simulink model "SMD_System"  (R2025b)
settings: Solver=VariableStepAuto  StartTime=0.0  StopTime=inf  MaxStep=0.01  RelTol=1e-3
undefined symbols (not defined in the file or in its folder): b
libraries: fl_lib x7, nesl_utility x3, fuzblock x1
settings Model: Creator=muham  LastModifiedBy=leffe
settings SolverCC: AlgebraicLoopSolver=TrustRegion
settings OptimizationCC: BlockReduction=off
settings DebuggingCC: UnconnectedInputMsg=warning  UnconnectedOutputMsg=warning  UnconnectedLineMsg=warning
settings ModelReferenceCC: EnableRefExpFcnMdlSchedulingChecks=on
settings SFSimCC: CustomCodeUndefinedFunction=UseInterfaceOnly
settings RTWCC: GPUComputeCapability=3.5
settings ExplorerConfigSet: SimMechanicsOpenEditorOnUpdate=off

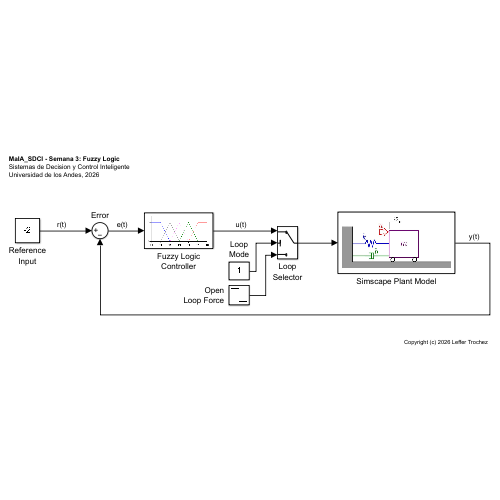
[thumbnail: Simulink's stored preview of the top-level diagram]
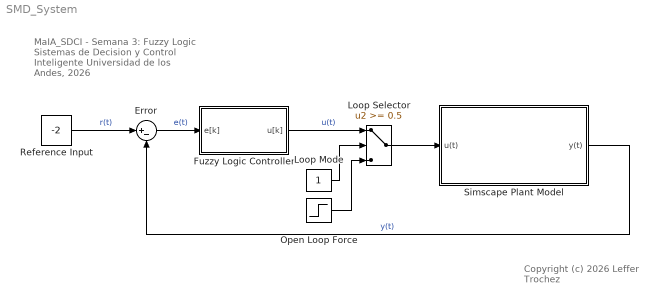
== system SMD_System ==
  note: Copyright (c) 2026 Leffer Trochez
  note: MaIA_SDCI - Semana 3: Fuzzy Logic
      | Sistemas de Decision y Control Inteligente
      | Universidad de los Andes, 2026
  Error : Sum  Inputs=|+-
  Fuzzy Logic Controller : Subsystem
      mask Display: image('fuzzy.png', [0,0,0,0,90,90]);
  Loop Mode : Constant
  Loop Selector : Switch  Threshold=0.5  SaturateOnIntegerOverflow=off  InputSameDT=off
  Open Loop Force : Step  Time=0.03  Before=500  After=0  SampleTime=0
  Reference Input : Constant  Value=-2  SampleTime=0
  Simscape Plant Model : Subsystem
      mask Display: image('Fig.png');
  wires:
  Error/1 -> Fuzzy Logic Controller/1(e[k])  "e(t)"
  Reference Input/1 -> Error/1  "r(t)"
  Simscape Plant Model/1(y(t)) -> Error/2  "y(t)"
  Fuzzy Logic Controller/1(u[k]) -> Loop Selector/1  "u(t)"
  Loop Mode/1 -> Loop Selector/2
  Open Loop Force/1 -> Loop Selector/3
  Loop Selector/1 -> Simscape Plant Model/1(u(t))

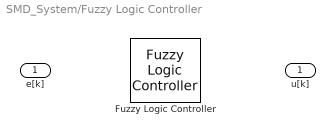
== system SMD_System/Fuzzy Logic Controller ==
  e[k] : Inport
  "Fuzzy Logic Controller " : fuzblock/Fuzzy Logic  Controller  FIS='tipper.fis'  OutputSampleNumber=101  DataType=double  UseLookupTable=off  NumBreakpoints=10  FuzzifiedInputs=off  RuleFiringStrengths=off  RuleOutputs=off  AggregatedOutputs=off  SimulateUsing=Interpreted execution  OutOfRangeInputValueMessage=warning  NoRuleFiredMessage=warning  EmptyOutputFuzzySetMessage=warning
  u[k] : Outport

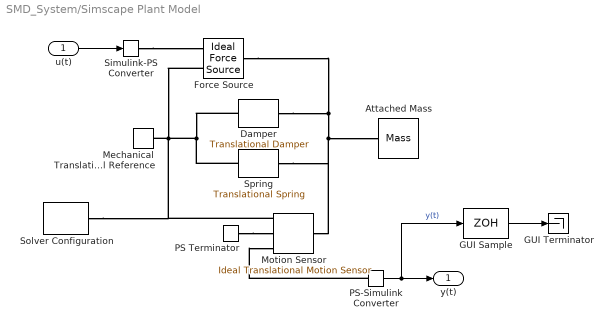
== system SMD_System/Simscape Plant Model ==
  u(t) : Inport
  Attached Mass : fl_lib/Mechanical/Translational Elements/Mass  mass=m kg  num_ports=foundation.enum.numPorts2.one  v_specify=off  v_priority=High  v=0 m/s  v_nominal_specify=off  v_nominal_value=1  v_nominal_unit=m/s  f_specify=off  f_priority=None  f=0 N  f_nominal_specify=off  f_nominal_value=1  f_nominal_unit=N
  Damper : fl_lib/Mechanical/Translational Elements/Translational Damper  D=b N/(m/s)  v_specify=off  v_priority=None  v=0 m/s  v_nominal_specify=off  v_nominal_value=1  v_nominal_unit=m/s  f_specify=off  f_priority=None  f=0 N  f_nominal_specify=off  f_nominal_value=1  f_nominal_unit=N
  Force Source : fl_lib/Mechanical/Mechanical Sources/Ideal Force Source
  GUI Terminator : Terminator
  GUI Sample : ZeroOrderHold  SampleTime=0.02
  Mechanical Translational Reference : fl_lib/Mechanical/Translational Elements/Mechanical Translational Reference
  Motion Sensor : fl_lib/Mechanical/Mechanical Sensors/Ideal Translational Motion Sensor  reference=foundation.enum.MeasurementReference.difference  acceleration_port=false  velocity_port=true  position_port=true  offset=0 m
  PS Terminator : fl_lib/Physical Signals/Sinks/PS Terminator
  PS-Simulink Converter : nesl_utility/PS-Simulink Converter  PhysicalDomain=network_engine_domain  SubClassName=ps_output  LeftPortType=input  RightPortType=output  PseudoPeriodic=off  Frequencies=[]  VectorFormat=1-D array  Unit=m  AffineConversion=off
  Simulink-PS Converter : nesl_utility/Simulink-PS Converter  PhysicalDomain=network_engine_domain  SubClassName=ps_input  LeftPortType=input  RightPortType=output  PseudoPeriodic=off  Frequencies=[]  NoiseDistribution=none  NoiseParameters=[]  Unit=N  AffineConversion=off  FilteringAndDerivatives=provide  SimscapeFilterOrder=1  InputFilterTimeConstant=0.001  UdotUserProvided=0
  Solver Configuration : nesl_utility/Solver Configuration  PhysicalDomain=network_engine_domain  SubClassName=solver  LeftPortType=input  RightPortType=generic  Tones=[]  Harmonics=[]  SimulateNoise=off  Profile=off  UseLocalSampling=off  EnableSwitchedLinearOptims=on  FrequencyDomain=off  UseCCode=off  RelTol=0.001  AbsTol=1e-06  MinStep=1e-09  ToWorkspace=off  RevertToSquareIcSolve=off  NumHomotopyIterations=100  PhasorMode=off  PhasorModeNumHarmonics=1  ConsistencySolver=NEWTON_FTOL  IndexReductionMethod=DerivativeReplacement  DoDC=off  ResidualTolerance=1e-09  ConsistencyTolSource=GLOBAL  ConsistencyAbsTol=0.001  ConsistencyRelTol=0.001  ConsistencyTolFactor=0.001  UseLocalSolver=off  LocalSolverChoice=NE_BACKWARD_EULER_ADVANCER  ResolveIndetEquations=on  FunctionEvalNumThread=1  LocalSolverSampleTime=0.001  DoFixedCost=off  MaxNonlinIter=3  MaxModeIter=2  ComputeImpulses=off  ImpulseIterations=2  LinearAlgebra=auto  LinearAlgebraNumThread=0  EquationFormulation=NE_TIME_EF  DelaysMemoryBudget=1024  AutomaticFiltering=on  FilteringTimeConstant=0.001  PartitionStorageMethod=AS_NEEDED  PartitionMemoryBudget=1024  PartitionMethod=ROBUST  MultibodyUseLocalSolver=off  MultibodyLocalSolverChoice=ODE1  MultibodyLocalSolverSampleTime=0.001
  Spring : fl_lib/Mechanical/Translational Elements/Translational Spring  spr_rate=k N/m  v_specify=off  v_priority=None  v=0 m/s  v_nominal_specify=off  v_nominal_value=1  v_nominal_unit=m/s  f_specify=off  f_priority=None  f=0 N  f_nominal_specify=off  f_nominal_value=1  f_nominal_unit=N  x_specify=off  x_priority=High  x=0 m  x_nominal_specify=off  x_nominal_value=1  x_nominal_unit=m
  y(t) : Outport  VectorParamsAs1DForOutWhenUnconnected=off
  wires:
  u(t)/1 -> Simulink-PS Converter/1
  GUI Sample/1 -> GUI Terminator/1
  PS-Simulink Converter/1 -> y(t)/1, GUI Sample/1  "y(t)"
  connections:
  Damper/LConn1 -- Force Source/LConn1 -- Motion Sensor/LConn1 -- Spring/LConn1 -- Attached Mass/LConn1
  Damper/RConn1 -- Spring/RConn1 -- Solver Configuration/RConn1 -- Motion Sensor/RConn1 -- Mechanical Translational Reference/LConn1 -- Force Source/RConn2
  PS Terminator/LConn1 -- Motion Sensor/RConn2
  PS-Simulink Converter/LConn1 -- Motion Sensor/RConn3
  Simulink-PS Converter/RConn1 -- Force Source/RConn1
